simulink model "Main_simulation_davide"  (R2021b)
settings: Solver=FixedStepAuto  StartTime=0.0  StopTime=Time  FixedStep=0.1  RelTol=1e-13  AbsTol=1e-19
values from neighbouring files (symbols this model uses):
  a = 8.6251e06    (= 8625100)    [main_code.m]
  A_BN_0 = eye(3)    [main_code.m]
  A_rw = [1 0 0 1/sqrt(3);         0 1 0 1/sqrt(3) ... (first row only)    [main_code.m]
  A_rw_star = [5/6 -1/6 -1/6;              -1/6  5/6 -1/6 ... (first row only)    [main_code.m]
  acc_m = deg2rad(5)    [main_code.m]
  acc_S = deg2rad(0.25)    [main_code.m]
  c = 2.99792*10^8    (= 299792000)    [main_code.m]
  control = 3    [main_code.m]
  e = 0.1195    [main_code.m]
  G = [gn, gm, gvali, gsvi]    [main_code.m]
  H = [hn, hm, hvali, hsvi]    [main_code.m]
  i = 0.3815    [main_code.m]
  MB = [1; 0.3; 0.3; 0.3]    [main_code.m]
  mr = 1.2*1e-4    (= 0.00012)    [main_code.m]
  mu_P = G * Mt    (= 398527110340000)    [main_code.m]
  omega_0 = [w_0x; w_0y; w_0z]    [main_code.m]
  rho_d_MB = 0.1    [main_code.m]
  rho_d_SP = 0.1    [main_code.m]
  rho_s_MB = 0.5    [main_code.m]
  rho_s_SP = 0.1    [main_code.m]
  sig_b = sig_b^2    [main_code.m]
  sig_n = 0.15*pi/180/3600/sqrt(t_sample)    [main_code.m]
  SP = [3; 0.3; 1; 0.1]    [main_code.m]
  t_sample = 1    [main_code.m]
  theta_0 = 0    [main_code.m]
undefined symbols (not defined in the file or in its folder): theta0
libraries: matrix_library x16, vrlib x10, simulink x3, simulink_extras x1
(part 2 of 4)

== system Main_simulation_davide/Attitude determination/Attitude determination/If Action Subsystem3 ==
  In1 : Inport
  Action Port : ActionPort  ActionPortLabel=if(u1 == u2)
  Out1 : Outport
  wires:
  In1/1 -> Out1/1

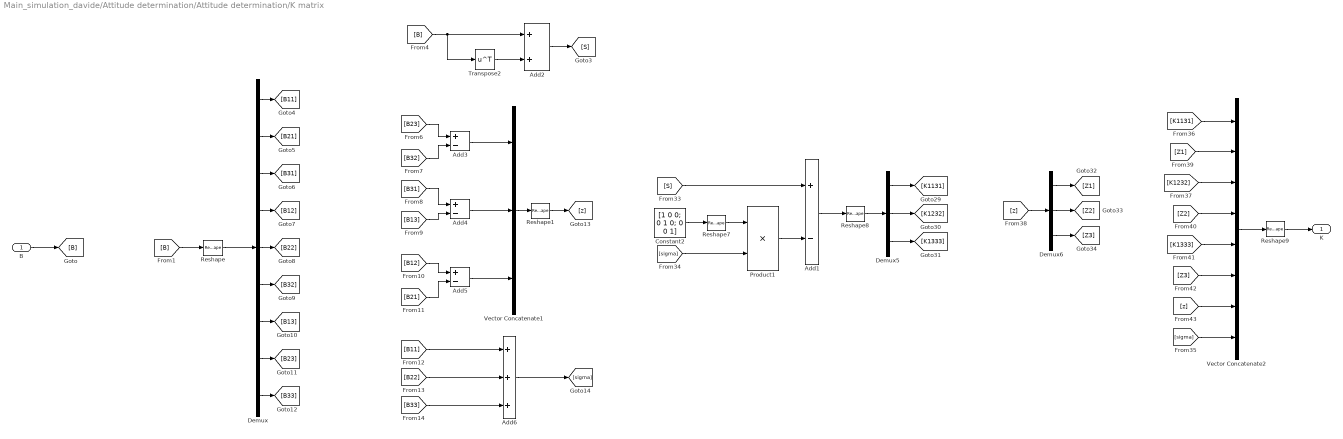
== system Main_simulation_davide/Attitude determination/Attitude determination/K matrix ==
  B : Inport
  Add{1,3..5} (4 alike) : Sum  Inputs=+-
  Add2 : Sum
  Add6 : Sum  Inputs=+++
  Constant2 : Constant  Value=[1 0 0; 0 1 0; 0 0 1]  VectorParams1D=off
  Demux : Demux  Outputs=9
  Demux5 : Demux  Outputs=3
  Demux6 : Demux  Outputs=3
  Product1 : Product
  Reshape : Reshape  OutputDimensionality=Column vector (2-D)
  Reshape1 : Reshape  OutputDimensionality=Column vector (2-D)
  Reshape7 : Reshape  OutputDimensionality=Customize  OutputDimensions=[3,3]
  Reshape8 : Reshape  OutputDimensionality=Column vector (2-D)
  Reshape9 : Reshape  OutputDimensionality=Customize  OutputDimensions=[4,4]
  Transpose2 : Math  Operator=transpose  SaturateOnIntegerOverflow=on
  Vector Concatenate1 : Concatenate  NumInputs=3
  Vector Concatenate2 : Concatenate  NumInputs=8
  K : Outport
  wires:
  Demux/9 -> [B33]
  Demux/3 -> [B31]
  Demux/5 -> [B22]
  Demux/2 -> [B21]
  Demux/8 -> [B23]
  Demux/7 -> [B13]
  Reshape/1 -> Demux/1
  Demux/6 -> [B32]
  Demux/1 -> [B11]
  Demux/4 -> [B12]
  Demux6/3 -> [Z3]
  [B21] -> Add5/2
  [B32] -> Add3/2
  [B33] -> Add6/3
  [B22] -> Add6/2
  [B23] -> Add3/1
  [B12] -> Add5/1
  Add4/1 -> Vector Concatenate1/2
  Transpose2/1 -> Add2/2
  Add5/1 -> Vector Concatenate1/3
  [B31] -> Add4/1
  Vector Concatenate1/1 -> Reshape1/1
  Reshape1/1 -> [z]
  Add6/1 -> [sigma]
  [B13] -> Add4/2
  [B11] -> Add6/1
  Add3/1 -> Vector Concatenate1/1
  [B] -> Transpose2/1, Add2/1
  Demux6/1 -> [Z1]
  Reshape8/1 -> Demux5/1
  Product1/1 -> Add1/2
  [S] -> Add1/1
  Constant2/1 -> Reshape7/1
  [sigma] -> Product1/2
  Add2/1 -> [S]
  Demux6/2 -> [Z2]
  Reshape7/1 -> Product1/1
  Demux5/2 -> [K1232]
  Demux5/3 -> [K1333]
  Demux5/1 -> [K1131]
  Add1/1 -> Reshape8/1
  [z] -> Demux6/1
  Vector Concatenate2/1 -> Reshape9/1
  [K1333] -> Vector Concatenate2/5
  [sigma] -> Vector Concatenate2/8
  [z] -> Vector Concatenate2/7
  [K1131] -> Vector Concatenate2/1
  [K1232] -> Vector Concatenate2/3
  [Z1] -> Vector Concatenate2/2
  [Z3] -> Vector Concatenate2/6
  [Z2] -> Vector Concatenate2/4
  Reshape9/1 -> K/1
  B/1 -> [B]
  [B] -> Reshape/1

== system Main_simulation_davide/Attitude determination/Attitude determination/q to DCM ==
  In1 : Inport
  Add : Sum  Inputs=+-
  Add1 : Sum  Inputs=++-
  Constant : Constant  Value=[1 0 0; 0 1 0; 0 0 1]  VectorParams1D=off
  Demux : Demux
  Gain : Gain  Gain=2
  Gain1 : Gain  Gain=2
  Matrix Multiply : Product  Multiplication=Matrix(*)
  Matrix Multiply2 : Product  Multiplication=Matrix(*)
  Mux : Mux  Inputs=3
  Product : Product
  Product1 : Product
  Reshape : Reshape  OutputDimensionality=Column vector (2-D)
  Reshape1 : Reshape  OutputDimensionality=Customize  OutputDimensions=[3,3]
  Square : Math  Operator=square  SaturateOnIntegerOverflow=on
  Transpose : Math  Operator=transpose  SaturateOnIntegerOverflow=on
  Transpose1 : Math  Operator=transpose  SaturateOnIntegerOverflow=on
  q_cross : Subsystem
  A_BN : Outport
  wires:
  In1/1 -> Demux/1
  Demux/4 -> [q4]
  Demux/1 -> [q1]
  Demux/2 -> [q2]
  Demux/3 -> [q3]
  [q4] -> Square/1
  [q2] -> Mux/2
  [q3] -> Mux/3
  [q1] -> Mux/1
  Mux/1 -> Reshape/1
  Reshape/1 -> [q_vect]
  [q_vect] -> Matrix Multiply/2, Transpose/1
  Transpose/1 -> Matrix Multiply/1
  Matrix Multiply/1 -> Add/2
  Square/1 -> Add/1
  Constant/1 -> Reshape1/1
  Reshape1/1 -> Product1/2
  Product1/1 -> Add1/1
  Matrix Multiply2/1 -> Gain/1
  Gain/1 -> Add1/2
  Transpose1/1 -> Matrix Multiply2/2
  [q_vect] -> Transpose1/1, Matrix Multiply2/1
  Gain1/1 -> Add1/3
  Product/1 -> Gain1/1
  [q4] -> Product/2
  q_cross/1(q_cross) -> Product/1
  Add1/1 -> A_BN/1
  [q_vect] -> q_cross/1(q_vect)
  Add/1 -> Product1/1

== system Main_simulation_davide/Attitude determination/Quaternion error/Q matrix ==
  q_eul : Inport
  Demux : Demux
  Gain{,1..5} (6 alike) : Gain  Gain=-1
  Reshape : Reshape  OutputDimensionality=Customize  OutputDimensions=[4,4]
  Vector Concatenate : Concatenate  NumInputs=16
  Q_eul : Outport
  wires:
  q_eul/1 -> Demux/1
  Demux/1 -> [q1]
  Demux/2 -> [q2]
  Demux/3 -> [q3]
  Demux/4 -> [q4]
  Reshape/1 -> Q_eul/1
  Vector Concatenate/1 -> Reshape/1
  [q4] -> Vector Concatenate/1
  [q3] -> Gain/1
  Gain/1 -> Vector Concatenate/2
  [q2] -> Vector Concatenate/3
  [q1] -> Vector Concatenate/4
  [q3] -> Vector Concatenate/5
  [q4] -> Vector Concatenate/6
  Gain1/1 -> Vector Concatenate/7
  [q1] -> Gain1/1
  [q2] -> Vector Concatenate/8
  [q2] -> Gain2/1
  Gain2/1 -> Vector Concatenate/9
  [q1] -> Vector Concatenate/10
  [q4] -> Vector Concatenate/11
  [q3] -> Vector Concatenate/12
  [q1] -> Gain3/1
  Gain4/1 -> Vector Concatenate/14
  Gain3/1 -> Vector Concatenate/13
  Gain5/1 -> Vector Concatenate/15
  [q2] -> Gain4/1
  [q3] -> Gain5/1
  [q4] -> Vector Concatenate/16

== system Main_simulation_davide/Attitude determination/Sensors/Gyroscopes ==
  note: gyro model: STIM300
  omega : Inport
  Integrator : Integrator
  Mux1 : Mux  Inputs=3
  Mux2 : Mux  Inputs=3
  Reshape : Reshape  OutputDimensionality=Column vector (2-D)
  Reshape1 : Reshape  OutputDimensionality=Column vector (2-D)
  Sum : Sum  Inputs=+++
  "b1 " : RandomNumber  Variance=sig_b  Seed=1  SampleTime=t_sample
  b2 : RandomNumber  Variance=sig_b  Seed=2  SampleTime=t_sample
  b3 : RandomNumber  Variance=sig_b  Seed=3  SampleTime=t_sample
  n1 : RandomNumber  Variance=sig_n  Seed=4  SampleTime=t_sample
  n2 : RandomNumber  Variance=sig_n  Seed=5  SampleTime=t_sample
  n3 : RandomNumber  Variance=sig_n  Seed=6  SampleTime=t_sample
  w_gyro : Outport
  wires:
  Integrator/1 -> Sum/1
  "b1 "/1 -> Mux1/1
  b2/1 -> Mux1/2
  b3/1 -> Mux1/3
  n3/1 -> Mux2/3
  n2/1 -> Mux2/2
  n1/1 -> Mux2/1
  Mux1/1 -> Reshape/1
  Mux2/1 -> Reshape1/1
  omega/1 -> Sum/2
  Reshape/1 -> Integrator/1
  Reshape1/1 -> Sum/3
  Sum/1 -> w_gyro/1

== system Main_simulation_davide/Attitude determination/Sensors/Magnetometer ==
  A_BN : Inport
  b_N : Inport  Port=2
  "Magnetometer " : Subsystem
  b_B computation : Subsystem
  model to reality difference : Subsystem
  b_B : Outport
  wires:
  "Magnetometer "/1(A_BN*_filtered) -> model to reality difference/2(A_BN*), b_B computation/1(A_BN*)
  A_BN/1 -> model to reality difference/1(A_BN), "Magnetometer "/1(A_BN)
  b_N/1 -> b_B computation/2(b_N), model to reality difference/3(b_N)
  b_B computation/1(b_B) -> b_B/1

== system Main_simulation_davide/Attitude determination/Sensors/Sun sensor ==
  note: redwire space, digital sun sensor +/- 64°
  S_N : Inport
  A_BN : Inport  Port=2
  Add : Sum  Inputs=+-
  Add1 : Sum  Inputs=+-
  Constant : Constant  Value=0.25*pi/180
  Constant1 : Constant
  Constant2 : Constant  Value=0.25*pi/180
  Constant3 : Constant  Value=0.25*pi/180
  Discrete Derivative : simulink/Discrete/Discrete Derivative  gainval=1e4  ICPrevScaledInput=0.0  OutMin=[]  OutMax=[]  OutDataType=fixdt(1, 16)  OutScaling=2^-10  DoSatur=off
  Gain : Gain  Gain=-1
  Gain1 : Gain  Gain=-1
  Gain2 : Gain  Gain=-1
  Matrix Multiply : Product  Multiplication=Matrix(*)
  Matrix Multiply1 : Product  Multiplication=Matrix(*)
  Product : Product
  Product1 : Product
  Product2 : Product
  Random Number : RandomNumber  Variance=0.6*pi/180  SampleTime=t_sample
  Random Number1 : RandomNumber  Variance=0.6*pi/180  SampleTime=t_sample
  Random Number2 : RandomNumber  Variance=0.6*pi/180  SampleTime=t_sample
  Reshape : Reshape  OutputDimensionality=Customize  OutputDimensions=[3,3]
  Scope : Scope
  Vector Concatenate : Concatenate  NumInputs=9
  S_B : Outport
  wires:
  S_N/1 -> Matrix Multiply1/2
  Random Number/1 -> Product/2
  Constant/1 -> Product/1
  Matrix Multiply/1 -> Add1/1
  Add1/1 -> Add/1, Discrete Derivative/1, S_B/1
  Constant1/1 -> Vector Concatenate/8, Vector Concatenate/5, Vector Concatenate/1
  Constant2/1 -> Product1/1
  Random Number1/1 -> Product1/2
  Random Number2/1 -> Product2/2
  Constant3/1 -> Product2/1
  Product2/1 -> Vector Concatenate/4, Gain/1
  Gain/1 -> Vector Concatenate/2
  Product1/1 -> Vector Concatenate/3, Gain2/1
  Gain1/1 -> Vector Concatenate/6
  Product/1 -> Gain1/1, Vector Concatenate/9
  Gain2/1 -> Vector Concatenate/7
  Discrete Derivative/1 -> Add1/2
  Reshape/1 -> Matrix Multiply/1
  Vector Concatenate/1 -> Reshape/1
  A_BN/1 -> Matrix Multiply1/1
  Matrix Multiply1/1 -> Add/2, Matrix Multiply/2
  Add/1 -> Scope/1

== system Main_simulation_davide/Control/Slew/Desired attitude ==
  S_N : Inport
  Constant : Constant  Value=0
  Constant1 : Constant
  Constant2 : Constant  Value=0
  Cross Product : matrix_library/Cross Product
      settings: SourceProductBaseCode=SL
  Display : Display
  Display1 : Display
  Dot Product : DotProduct  InputSameDT=on  OutDataTypeStr=Inherit: Inherit via internal rule
  Matrix Multiply : Product  Multiplication=Matrix(*)
  Mux : Mux  Inputs=3
  Reshape : Reshape  OutputDimensionality=Column vector (2-D)
  Reshape1 : Reshape  OutputDimensionality=Customize  OutputDimensions=[3,3]
  Transpose : Math  Operator=transpose  SaturateOnIntegerOverflow=on
  Transpose1 : Math  Operator=transpose  SaturateOnIntegerOverflow=on
  Vector Concatenate : Concatenate  NumInputs=3
  orthonormalization step 1 : Subsystem
  Desired A_BN : Outport
  wires:
  Constant/1 -> Mux/1
  Constant1/1 -> Mux/2
  Constant2/1 -> Mux/3
  Mux/1 -> Reshape/1
  Reshape/1 -> Vector Concatenate/2, Cross Product/2
  S_N/1 -> Dot Product/2, Dot Product/1, Vector Concatenate/1, Cross Product/1
  Vector Concatenate/1 -> Reshape1/1
  Reshape1/1 -> Transpose/1
  Transpose1/1 -> Matrix Multiply/2
  Matrix Multiply/1 -> Display/1
  Dot Product/1 -> Display1/1
  Transpose/1 -> orthonormalization step 1/1(A*(t))
  orthonormalization step 1/1(A_BN*_filtered) -> Transpose1/1, Matrix Multiply/1, Desired A_BN/1
  Cross Product/1 -> Vector Concatenate/3

== system Main_simulation_davide/Control/Slew/Reaction wheel ==
  Mc : Inport
  w : Inport  Port=2
  A : Constant  Value=A_rw
  A_star : Constant  Value=A_rw_star
  Add : Sum  Inputs=--
  Constant : Constant  Value=[0 0 0 0]
  Cross Product : matrix_library/Cross Product
      settings: SourceProductBaseCode=SL
  Cross Product1 : matrix_library/Cross Product
      settings: SourceProductBaseCode=SL
  Gain : Gain  Gain=-1
  Integrator : Integrator  InitialConditionSource=external
  Matrix Multiply{,1..3} (4 alike) : Product  Multiplication=Matrix(*)
  Reshape : Reshape  OutputDimensionality=Column vector (2-D)
  Reshape1 : Reshape  OutputDimensionality=Column vector (2-D)
  Sum : Sum  Inputs=|++
  Mr : Outport
  wires:
  Cross Product1/1 -> Add/2
  [h_r] -> Matrix Multiply3/2
  [A_rw] -> Matrix Multiply3/1
  Matrix Multiply3/1 -> Cross Product1/2
  [omega] -> Cross Product1/1
  Add/1 -> Mr/1
  Matrix Multiply2/1 -> Add/1
  [A_rw] -> Matrix Multiply2/1
  Reshape1/1 -> Sum/2
  Reshape/1 -> Integrator/2
  Constant/1 -> Reshape/1
  Matrix Multiply1/1 -> Matrix Multiply2/2, Integrator/1
  Gain/1 -> Matrix Multiply1/1
  A_star/1 -> Gain/1
  Sum/1 -> Matrix Multiply1/2
  Mc/1 -> Reshape1/1
  Cross Product/1 -> Sum/1
  Matrix Multiply/1 -> Cross Product/2
  w/1 -> Cross Product/1, [omega]
  A/1 -> Matrix Multiply/1, [A_rw]
  Integrator/1 -> Matrix Multiply/2, [h_r]

== system Main_simulation_davide/Control/Target tracking/Reaction wheel ==
  Mc : Inport
  w : Inport  Port=2
  A : Constant  Value=A_rw
  A_star : Constant  Value=A_rw_star
  Add : Sum  Inputs=--
  Constant : Constant  Value=[0 0 0 0]
  Cross Product : matrix_library/Cross Product
      settings: SourceProductBaseCode=SL
  Cross Product1 : matrix_library/Cross Product
      settings: SourceProductBaseCode=SL
  Gain : Gain  Gain=-1
  Integrator : Integrator  InitialConditionSource=external
  Matrix Multiply{,1..3} (4 alike) : Product  Multiplication=Matrix(*)
  Reshape : Reshape  OutputDimensionality=Column vector (2-D)
  Reshape1 : Reshape  OutputDimensionality=Column vector (2-D)
  Sum : Sum  Inputs=|++
  Mr : Outport
  wires:
  Cross Product1/1 -> Add/2
  [h_r] -> Matrix Multiply3/2
  [A_rw] -> Matrix Multiply3/1
  Matrix Multiply3/1 -> Cross Product1/2
  [omega] -> Cross Product1/1
  Add/1 -> Mr/1
  Matrix Multiply2/1 -> Add/1
  [A_rw] -> Matrix Multiply2/1
  Reshape1/1 -> Sum/2
  Reshape/1 -> Integrator/2
  Constant/1 -> Reshape/1
  Matrix Multiply1/1 -> Matrix Multiply2/2, Integrator/1
  Gain/1 -> Matrix Multiply1/1
  A_star/1 -> Gain/1
  Sum/1 -> Matrix Multiply1/2
  Mc/1 -> Reshape1/1
  Cross Product/1 -> Sum/1
  Matrix Multiply/1 -> Cross Product/2
  w/1 -> Cross Product/1, [omega]
  A/1 -> Matrix Multiply/1, [A_rw]
  Integrator/1 -> Matrix Multiply/2, [h_r]

== system Main_simulation_davide/Enviroment/Magnetic field/b_B ==
  A_BN : Inport
  R : Inport  Port=2
  r_LVLH : Inport  Port=3
  Clock : Clock
  Constant3 : Constant  Value=G
  Constant4 : Constant  Value=H
  MATLAB Function : MATLAB Function  TreatAsAtomicUnit=on
  MatrixMultiply : Product  Multiplication=Matrix(*)
  Reshape1 : Reshape  OutputDimensionality=Column vector (2-D)
  b_B : Outport
  b_N : Outport  Port=2
  wires:
  MatrixMultiply/1 -> b_B/1
  A_BN/1 -> [A_BN]
  [A_BN] -> MatrixMultiply/1
  r_LVLH/1 -> MATLAB Function/1(r_LVLH)
  R/1 -> MATLAB Function/2(r)
  Clock/1 -> MATLAB Function/3(t)
  MATLAB Function/1(b_N) -> Reshape1/1
  Constant3/1 -> MATLAB Function/4(G)
  Constant4/1 -> MATLAB Function/5(H)
  Reshape1/1 -> b_N/1, MatrixMultiply/2

== system Main_simulation_davide/Enviroment/Magnetic field/parasitic torque ==
  Constant : Constant  Value=0.01
  Constant1 : Constant  Value=0.05
  Constant2 : Constant  Value=0.01
  Mux : Mux  Inputs=3
  Reshape : Reshape  OutputDimensionality=Column vector (2-D)
  m_par : Outport
  wires:
  Constant/1 -> Mux/1
  Constant1/1 -> Mux/2
  Constant2/1 -> Mux/3
  Mux/1 -> Reshape/1
  Reshape/1 -> m_par/1

== system Main_simulation_davide/Enviroment/Solar radiation/Areas ==
  MB : Inport
  Demux : Demux
  Mux : Mux  Inputs=3
  Product1 : Product
  Product2 : Product
  Product4 : Product
  Terminator : Terminator
  A_vect : Outport
  wires:
  Product2/1 -> Mux/2  "a*h"
  Product4/1 -> Mux/1  "b*h"
  MB/1 -> Demux/1
  Product1/1 -> Mux/3  "a*b"
  Demux/1 -> Terminator/1
  Demux/2 -> [a]
  Demux/3 -> [b]
  Demux/4 -> [h]
  [b] -> Product4/1
  [h] -> Product4/2
  [h] -> Product2/2
  [b] -> Product1/2
  [a] -> Product2/1
  [a] -> Product1/1
  Mux/1 -> A_vect/1

== system Main_simulation_davide/Enviroment/Solar radiation/Areas_SP ==
  SP : Inport
  Demux : Demux
  Product1 : Product
  Terminator : Terminator
  Terminator1 : Terminator
  A_vect : Outport
  wires:
  [a] -> Product1/1
  [b] -> Product1/2
  Demux/4 -> Terminator1/1
  Demux/3 -> [b]
  Demux/2 -> [a]
  Demux/1 -> Terminator/1
  Product1/1 -> A_vect/1  "a*b"
  SP/1 -> Demux/1

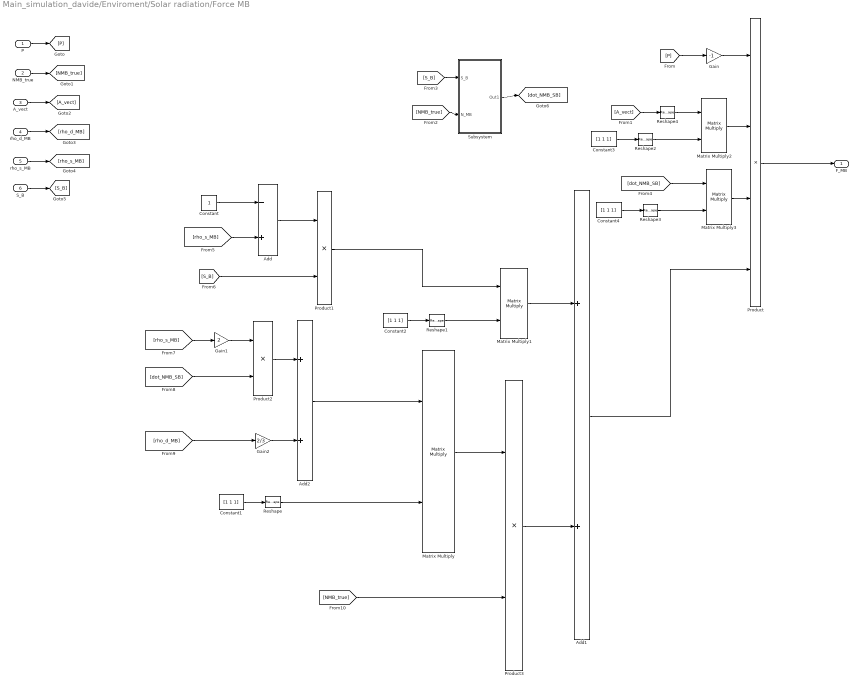
== system Main_simulation_davide/Enviroment/Solar radiation/Force MB ==
  P : Inport
  NMB_true : Inport  Port=2
  A_vect : Inport  Port=3
  rho_d_MB : Inport  Port=4
  rho_s_MB : Inport  Port=5
  S_B : Inport  Port=6
  Add : Sum  Inputs=-+
  Add1 : Sum
  Add2 : Sum
  Constant : Constant
  Constant{1..4} (4 alike) : Constant  Value=[1 1 1]
  Gain : Gain  Gain=-1
  Gain1 : Gain  Gain=2
  Gain2 : Gain  Gain=2/3
  Matrix Multiply{,1..3} (4 alike) : Product  Multiplication=Matrix(*)
  Product : Product  Inputs=4
  Product1 : Product
  Product2 : Product
  Product3 : Product
  Reshape{,1..3} (4 alike) : Reshape  OutputDimensionality=Row vector (2-D)
  Reshape4 : Reshape  OutputDimensionality=Column vector (2-D)
  Subsystem : Subsystem
  F_MB : Outport
  wires:
  Product/1 -> F_MB/1
  P/1 -> [P]
  NMB_true/1 -> [NMB_true]
  A_vect/1 -> [A_vect]
  rho_d_MB/1 -> [rho_d_MB]
  rho_s_MB/1 -> [rho_s_MB]
  S_B/1 -> [S_B]
  [P] -> Gain/1
  Gain/1 -> Product/1
  [NMB_true] -> Subsystem/2(N_MB)
  [S_B] -> Subsystem/1(S_B)
  Subsystem/1(Out1) -> [dot_NMB_SB]
  [rho_s_MB] -> Add/2
  Constant/1 -> Add/1
  Add/1 -> Product1/1
  [S_B] -> Product1/2
  [rho_s_MB] -> Gain1/1
  [dot_NMB_SB] -> Product2/2
  Gain1/1 -> Product2/1
  Product2/1 -> Add2/1
  Gain2/1 -> Add2/2
  [rho_d_MB] -> Gain2/1
  [NMB_true] -> Product3/2
  Product3/1 -> Add1/2
  Add1/1 -> Product/4
  Constant1/1 -> Reshape/1
  Matrix Multiply/1 -> Product3/1
  Add2/1 -> Matrix Multiply/1
  Reshape/1 -> Matrix Multiply/2
  Matrix Multiply1/1 -> Add1/1
  Product1/1 -> Matrix Multiply1/1
  Constant2/1 -> Reshape1/1
  Reshape1/1 -> Matrix Multiply1/2
  Reshape2/1 -> Matrix Multiply2/2
  Constant3/1 -> Reshape2/1
  Reshape3/1 -> Matrix Multiply3/2
  Constant4/1 -> Reshape3/1
  [A_vect] -> Reshape4/1
  Reshape4/1 -> Matrix Multiply2/1
  [dot_NMB_SB] -> Matrix Multiply3/1
  Matrix Multiply3/1 -> Product/3
  Matrix Multiply2/1 -> Product/2

== system Main_simulation_davide/Enviroment/Solar radiation/Force SP ==
  P : Inport
  NSP_true : Inport  Port=2
  A_vect_SP : Inport  Port=3
  rho_d_SP : Inport  Port=4
  rho_s_SP : Inport  Port=5
  S_B : Inport  Port=6
  Add : Sum  Inputs=+-
  Add1 : Sum
  Add2 : Sum
  Constant : Constant
  Dot Product : DotProduct  InputSameDT=on  OutDataTypeStr=Inherit: Inherit via internal rule
  Dot Product1 : DotProduct  InputSameDT=on  OutDataTypeStr=Inherit: Inherit via internal rule
  Gain : Gain  Gain=-1
  Gain1 : Gain  Gain=2
  Gain2 : Gain  Gain=2/3
  Product : Product  Inputs=4
  Product1 : Product
  Product2 : Product
  Product3 : Product
  Reshape : Reshape  OutputDimensionality=Row vector (2-D)
  Transpose : Math  Operator=transpose  SaturateOnIntegerOverflow=on
  F_SP : Outport
  wires:
  P/1 -> [P]
  NSP_true/1 -> [NSP_true]
  A_vect_SP/1 -> [A_vect_SP]
  rho_d_SP/1 -> [rho_d_SP]
  rho_s_SP/1 -> [rho_s_SP]
  S_B/1 -> [S_B]
  Product/1 -> Reshape/1
  [P] -> Gain/1
  Gain/1 -> Product/1
  [A_vect_SP] -> Product/2
  Dot Product/1 -> Product/3
  [S_B] -> Dot Product/2
  [NSP_true] -> Dot Product/1
  Constant/1 -> Add/1
  [rho_s_SP] -> Add/2
  Add/1 -> Product1/1
  [S_B] -> Product1/2
  [rho_s_SP] -> Gain1/1
  [NSP_true] -> Dot Product1/1
  [S_B] -> Dot Product1/2
  Dot Product1/1 -> Product2/2
  Gain1/1 -> Product2/1
  Product2/1 -> Add1/1
  [rho_d_SP] -> Gain2/1
  Gain2/1 -> Add1/2
  [NSP_true] -> Transpose/1
  Add1/1 -> Product3/1
  Product1/1 -> Add2/1
  Product3/1 -> Add2/2
  Transpose/1 -> Product3/2
  Add2/1 -> Product/4
  Reshape/1 -> F_SP/1

== system Main_simulation_davide/Enviroment/Solar radiation/Pressure ==
  Constant6 : Constant  Value=1358
  Constant7 : Constant  Value=c
  Product8 : Product
  Reciprocal : Product  Inputs=/
  P : Outport
  wires:
  Constant6/1 -> Product8/1
  Reciprocal/1 -> Product8/2
  Product8/1 -> P/1
  Constant7/1 -> Reciprocal/1

== system Main_simulation_davide/Enviroment/Solar radiation/S_B dot N_MB ==
  N_MB : Inport
  S_B : Inport  Port=2
  Constant3 : Constant  Value=[1, 1, 1, 1, 1, 1]  VectorParams1D=off
  Demux : Demux  Outputs=6
  If : If
  If Action Subsystem : Subsystem  TreatAsAtomicUnit=on
  If Action Subsystem1 : Subsystem  TreatAsAtomicUnit=on
  If Action Subsystem2 : Subsystem  TreatAsAtomicUnit=on
  If Action Subsystem3 : Subsystem  TreatAsAtomicUnit=on
  If Action Subsystem4 : Subsystem  TreatAsAtomicUnit=on
  If Action Subsystem5 : Subsystem  TreatAsAtomicUnit=on
  If1 : If
  If2 : If
  Matrix Multiply5 : Product  Multiplication=Matrix(*)
  Merge{,1..5} (6 alike) : Merge
  Mux : Mux  Inputs=3
  Product10 : Product
  Reshape{,1..4,12} (6 alike) : Reshape  OutputDimensionality=Column vector (2-D)
  Reshape11 : Reshape  OutputDimensionality=Row vector (2-D)
  Reshape5 : Reshape  OutputDimensionality=Customize  OutputDimensions=[3,3]
  Sum of Elements : Sum  Inputs=+  CollapseMode=Specified dimension  CollapseDim=2
  Terminator1 : Terminator
  Terminator2 : Terminator
  Terminator3 : Terminator
  Transpose : Math  Operator=transpose  SaturateOnIntegerOverflow=on
  Vector Concatenate : Concatenate  NumInputs=3
  MB_illuminated : Outport
  pointer : Outport  Port=2
  wires:
  Reshape12/1 -> Matrix Multiply5/1
  Matrix Multiply5/1 -> Transpose/1
  Product10/1 -> Sum of Elements/1
  Reshape11/1 -> Matrix Multiply5/2
  Constant3/1 -> Reshape11/1
  S_B/1 -> Reshape12/1
  Sum of Elements/1 -> Reshape/1
  Reshape/1 -> Demux/1
  Demux/1 -> If/1
  If/1 -> If Action Subsystem/Action
  If/2 -> If Action Subsystem3/Action
  N_MB/1 -> [N_MB]
  [N_MB] -> Product10/2
  [N_MB] -> If Action Subsystem/1(NMB)
  Demux/4 -> Terminator1/1
  Demux/5 -> Terminator2/1
  Demux/6 -> Terminator3/1
  Demux/2 -> If1/1
  If1/1 -> If Action Subsystem1/Action
  [N_MB] -> If Action Subsystem3/1(NMB)
  [N_MB] -> If Action Subsystem1/1(NMB)
  If1/2 -> If Action Subsystem4/Action
  [N_MB] -> If Action Subsystem4/1(NMB)
  If Action Subsystem3/1(-x) -> Merge/2
  If Action Subsystem/1(x) -> Merge/1
  If Action Subsystem1/1(y) -> Merge1/1
  If Action Subsystem2/1(z) -> Merge2/1
  If Action Subsystem5/1(-z) -> Merge2/2
  Demux/3 -> If2/1
  If2/1 -> If Action Subsystem2/Action
  If2/2 -> If Action Subsystem5/Action
  [N_MB] -> If Action Subsystem2/1(NMB)
  [N_MB] -> If Action Subsystem5/1(NMB)
  Merge/1 -> Reshape1/1
  Merge1/1 -> Reshape2/1
  Merge2/1 -> Reshape3/1
  Reshape1/1 -> Vector Concatenate/1
  Reshape2/1 -> Vector Concatenate/2
  Reshape3/1 -> Vector Concatenate/3
  Vector Concatenate/1 -> Reshape5/1
  If Action Subsystem4/1(-y) -> Merge1/2
  If Action Subsystem/2(pointer) -> Merge4/1
  If Action Subsystem3/2(pointer) -> Merge4/2
  If Action Subsystem1/2(pointer) -> Merge5/1
  If Action Subsystem4/2(pointer) -> Merge5/2
  If Action Subsystem2/2(pointer) -> Merge3/1
  If Action Subsystem5/2(pointer) -> Merge3/2
  Merge4/1 -> Mux/1
  Merge5/1 -> Mux/2
  Merge3/1 -> Mux/3
  Mux/1 -> Reshape4/1
  Reshape4/1 -> pointer/1
  Reshape5/1 -> MB_illuminated/1
  Transpose/1 -> Product10/1

== system Main_simulation_davide/Enviroment/Solar radiation/S_B dot N_SP ==
  N_SP : Inport
  S_B : Inport  Port=2
  Constant3 : Constant  Value=[1, 1]
  Demux : Demux  Outputs=2
  If : If
  If Action Subsystem : Subsystem  TreatAsAtomicUnit=on
  If Action Subsystem1 : Subsystem  TreatAsAtomicUnit=on
  If1 : If
  Matrix Multiply5 : Product  Multiplication=Matrix(*)
  Merge : Merge
  Merge1 : Merge
  Product10 : Product
  Reshape11 : Reshape  OutputDimensionality=Row vector (2-D)
  Reshape12 : Reshape  OutputDimensionality=Column vector (2-D)
  Sum of Elements : Sum  Inputs=+  CollapseMode=Specified dimension  CollapseDim=2
  Terminator : Terminator
  Terminator1 : Terminator
  Transpose : Math  Operator=transpose  SaturateOnIntegerOverflow=on
  SP_illuminated : Outport
  pointer : Outport  Port=2
  wires:
  [N_SP] -> Product10/2
  N_SP/1 -> [N_SP]
  Sum of Elements/1 -> Demux/1
  S_B/1 -> Reshape12/1
  Constant3/1 -> Reshape11/1
  Reshape11/1 -> Matrix Multiply5/2
  Product10/1 -> Sum of Elements/1
  Matrix Multiply5/1 -> Transpose/1
  Reshape12/1 -> Matrix Multiply5/1
  Transpose/1 -> Product10/1
  Demux/1 -> If/1
  If/1 -> If Action Subsystem/Action
  Demux/2 -> If1/1
  [N_SP] -> If Action Subsystem/1(N_SP)
  [N_SP] -> If Action Subsystem1/1(N_SP)
  If1/1 -> If Action Subsystem1/Action
  If1/2 -> Terminator/1
  If/2 -> Terminator1/1
  If Action Subsystem/1(true_NSP) -> Merge/1
  If Action Subsystem1/1(true_NSP) -> Merge/2
  If Action Subsystem/2(pointer) -> Merge1/1
  If Action Subsystem1/2(pointer) -> Merge1/2
  Merge/1 -> SP_illuminated/1
  Merge1/1 -> pointer/1

== system Main_simulation_davide/Enviroment/Solar radiation/Sun position ==
  A_B_N : Inport
  Clock : Clock
  Constant : Constant  Value=2*pi
  Constant1 : Constant  Value=365*24*60*60
  Constant2 : Constant  Value=23.45
  Degrees to Radians : simulink_extras/Transformations/Degrees to Radians
  MatrixMultiply : Product  Multiplication=Matrix(*)
  Mux : Mux  Inputs=3
  Product{,1..3} (4 alike) : Product
  Reciprocal : Product  Inputs=1
  Reshape : Reshape  OutputDimensionality=Column vector (2-D)
  Sin : Trigonometry  Operator=cos
  Sin1 : Trigonometry
  Sin2 : Trigonometry  Operator=cos
  Sin3 : Trigonometry
  S_B : Outport
  S_N : Outport  Port=2
  wires:
  Product3/1 -> Mux/3
  Degrees to Radians/1 -> Sin3/1, Sin2/1
  Constant1/1 -> Reciprocal/1
  Sin2/1 -> Product2/2
  Product/1 -> Product1/1  "n"
  Constant2/1 -> Degrees to Radians/1
  Product1/1 -> Sin/1, Sin1/1  "n*t"
  Product2/1 -> Mux/2
  Sin3/1 -> Product3/2
  Clock/1 -> Product1/2
  Sin1/1 -> Product3/1, Product2/1
  Constant/1 -> Product/1
  Sin/1 -> Mux/1
  Reciprocal/1 -> Product/2
  Mux/1 -> Reshape/1
  A_B_N/1 -> MatrixMultiply/1
  MatrixMultiply/1 -> S_B/1
  Reshape/1 -> S_N/1, MatrixMultiply/2

== system Main_simulation_davide/Enviroment/Solar radiation/Torque arm MB ==
  note: creo il vettore somma che ha per colonna i raggi vettori che collegano il CM del MB con i centri illuminati delle facce nel caso che il sole sia nelle 4 posizioni.
  MB : Inport
  A_vect : Inport  Port=2
  S_B : Inport  Port=3
  pointer : Inport  Port=4
  Demux : Demux  Outputs=3
  Reshape : Reshape  OutputDimensionality=Customize  OutputDimensions=[3,3]
  Transpose : Math  Operator=transpose  SaturateOnIntegerOverflow=on
  Vector Concatenate : Concatenate  NumInputs=3
  creazione raggi vettore tra CM MB e centro facce illuminate della faccia che ha come normale l'asse i : Subsystem
  creazione raggi vettore tra CM MB e centro facce illuminate della faccia che ha come normale l'asse j : Subsystem
  creazione raggi vettore tra CM MB e centro facce illuminate della faccia che ha come normale l'asse k : Subsystem
  dist : Outport
  wires:
  pointer/1 -> Demux/1
  [x] -> creazione raggi vettore tra CM MB e centro facce illuminate della faccia che ha come normale l'asse i/4(pointer)
  [A_vect] -> creazione raggi vettore tra CM MB e centro facce illuminate della faccia che ha come normale l'asse i/3(A_vect)
  [MB] -> creazione raggi vettore tra CM MB e centro facce illuminate della faccia che ha come normale l'asse k/2(MB)
  [y] -> creazione raggi vettore tra CM MB e centro facce illuminate della faccia che ha come normale l'asse j/4(pointer)
  S_B/1 -> [S_B]
  [A_vect] -> creazione raggi vettore tra CM MB e centro facce illuminate della faccia che ha come normale l'asse k/3(A_vect)
  [MB] -> creazione raggi vettore tra CM MB e centro facce illuminate della faccia che ha come normale l'asse j/2(MB)
  A_vect/1 -> [A_vect]
  MB/1 -> [MB]
  [MB] -> creazione raggi vettore tra CM MB e centro facce illuminate della faccia che ha come normale l'asse i/2(MB)
  Reshape/1 -> Transpose/1
  Transpose/1 -> dist/1
  [S_B] -> creazione raggi vettore tra CM MB e centro facce illuminate della faccia che ha come normale l'asse k/1(S_B)
  Demux/1 -> [x]
  Demux/3 -> [z]
  [S_B] -> creazione raggi vettore tra CM MB e centro facce illuminate della faccia che ha come normale l'asse j/1(S_B)
  [z] -> creazione raggi vettore tra CM MB e centro facce illuminate della faccia che ha come normale l'asse k/4(pointer)
  Vector Concatenate/1 -> Reshape/1  "vectors x, y, z"
  [A_vect] -> creazione raggi vettore tra CM MB e centro facce illuminate della faccia che ha come normale l'asse j/3(A_vect)
  [S_B] -> creazione raggi vettore tra CM MB e centro facce illuminate della faccia che ha come normale l'asse i/1(S_B)
  Demux/2 -> [y]
  creazione raggi vettore tra CM MB e centro facce illuminate della faccia che ha come normale l'asse k/1(Out1) -> Vector Concatenate/3
  creazione raggi vettore tra CM MB e centro facce illuminate della faccia che ha come normale l'asse j/1(Out1) -> Vector Concatenate/2
  creazione raggi vettore tra CM MB e centro facce illuminate della faccia che ha come normale l'asse i/1(Out1) -> Vector Concatenate/1

== system Main_simulation_davide/Enviroment/Solar radiation/Torque arm SP ==
  SP : Inport
  A_vect_SP : Inport  Port=2
  S_B : Inport  Port=3
  pointer_SP : Inport  Port=4
  r_SP1 : Inport  Port=5
  r_SP2 : Inport  Port=6
  Add : Sum
  Add1 : Sum
  Reshape : Reshape  OutputDimensionality=Customize  OutputDimensions=[2,3]
  Vector Concatenate : Concatenate
  creazione raggi vettore tra CM SP e centro facce illuminate della faccia che ha come normale l'asse j : Subsystem
  distance : Outport
  wires:
  Reshape/1 -> distance/1
  SP/1 -> [SP]
  A_vect_SP/1 -> [A_vect_SP]
  S_B/1 -> [S_B]
  pointer_SP/1 -> [pointer_SP]
  r_SP1/1 -> [r_SP1]
  r_SP2/1 -> [r_SP2]
  [S_B] -> creazione raggi vettore tra CM SP e centro facce illuminate della faccia che ha come normale l'asse j/1(S_B)
  [SP] -> creazione raggi vettore tra CM SP e centro facce illuminate della faccia che ha come normale l'asse j/2(SP)
  [A_vect_SP] -> creazione raggi vettore tra CM SP e centro facce illuminate della faccia che ha come normale l'asse j/3(A_vect)
  [pointer_SP] -> creazione raggi vettore tra CM SP e centro facce illuminate della faccia che ha come normale l'asse j/4(pointer)
  creazione raggi vettore tra CM SP e centro facce illuminate della faccia che ha come normale l'asse j/1(distance) -> [distance]
  Vector Concatenate/1 -> Reshape/1
  Add/1 -> Vector Concatenate/1
  [distance] -> Add/1
  [r_SP1] -> Add/2
  [r_SP2] -> Add1/2
  [distance] -> Add1/1
  Add1/1 -> Vector Concatenate/2

== system Main_simulation_davide/Kinematics/DCM to quaternion/Case 1 ==
  A11 : Inport
  A22 : Inport  Port=2
  A33 : Inport  Port=3
  Add : Sum  Inputs=++--
  Constant : Constant
  Gain : Gain  Gain=1/2
  Sqrt : Sqrt  SaturateOnIntegerOverflow=on
  q1 : Outport
  wires:
  A22/1 -> Add/3
  A11/1 -> Add/2
  A33/1 -> Add/4
  Constant/1 -> Add/1
  Add/1 -> Sqrt/1
  Sqrt/1 -> Gain/1
  Gain/1 -> q1/1

== system Main_simulation_davide/Kinematics/DCM to quaternion/Case 2 ==
  A11 : Inport
  A22 : Inport  Port=2
  A33 : Inport  Port=3
  Add : Sum  Inputs=+-+-
  Constant : Constant
  Gain : Gain  Gain=1/2
  Sqrt : Sqrt  SaturateOnIntegerOverflow=on
  q2 : Outport
  wires:
  Gain/1 -> q2/1
  Sqrt/1 -> Gain/1
  Add/1 -> Sqrt/1
  Constant/1 -> Add/1
  A33/1 -> Add/4
  A11/1 -> Add/2
  A22/1 -> Add/3

== system Main_simulation_davide/Kinematics/DCM to quaternion/Case 3 ==
  A11 : Inport
  A22 : Inport  Port=2
  A33 : Inport  Port=3
  Add : Sum  Inputs=+--+
  Constant : Constant
  Gain : Gain  Gain=1/2
  Sqrt : Sqrt  SaturateOnIntegerOverflow=on
  q3 : Outport
  wires:
  A22/1 -> Add/3
  A11/1 -> Add/2
  A33/1 -> Add/4
  Constant/1 -> Add/1
  Add/1 -> Sqrt/1
  Sqrt/1 -> Gain/1
  Gain/1 -> q3/1

== system Main_simulation_davide/Kinematics/DCM to quaternion/Case 4 ==
  A11 : Inport
  A22 : Inport  Port=2
  A33 : Inport  Port=3
  Add : Sum  Inputs=++++
  Constant : Constant
  Gain : Gain  Gain=1/2
  Sqrt : Sqrt  SaturateOnIntegerOverflow=on
  q4 : Outport
  wires:
  Gain/1 -> q4/1
  Sqrt/1 -> Gain/1
  Add/1 -> Sqrt/1
  Constant/1 -> Add/1
  A33/1 -> Add/4
  A11/1 -> Add/2
  A22/1 -> Add/3

== system Main_simulation_davide/Kinematics/DCM to quaternion/If Action Subsystem ==
  In2 : Inport
  In1 : Inport  Port=2
  Action Port : ActionPort  ActionPortLabel=if(u1 == u2)
  Add : Sum
  Add1 : Sum
  Add2 : Sum  Inputs=+-
  Demux : Demux  Outputs=6
  Gain : Gain  Gain=4
  Mux : Mux
  Product : Product
  Product1 : Product
  Product2 : Product
  Reciprocal : Product  Inputs=/
  Reshape : Reshape  OutputDimensionality=Column vector (2-D)
  q_vect1 : Outport
  wires:
  In1/1 -> Demux/1
  In2/1 -> [q1]
  Mux/1 -> Reshape/1
  Reshape/1 -> q_vect1/1
  [q1] -> Mux/1
  Demux/3 -> [A12]
  Demux/2 -> [A31]
  Demux/1 -> [A21]
  Demux/6 -> [A23]
  Demux/5 -> [A13]
  Demux/4 -> [A32]
  [q1] -> Gain/1
  Gain/1 -> Reciprocal/1
  Reciprocal/1 -> [q1_div]
  Add/1 -> Product/1
  [A21] -> Add/2
  [A12] -> Add/1
  [q1_div] -> Product/2
  Product/1 -> [q2]
  Product1/1 -> [q3]
  [q1_div] -> Product1/2
  [A13] -> Add1/1
  [A31] -> Add1/2
  Add1/1 -> Product1/1
  Add2/1 -> Product2/1
  [A32] -> Add2/2
  [A23] -> Add2/1
  [q1_div] -> Product2/2
  Product2/1 -> [q4]
  [q2] -> Mux/2
  [q3] -> Mux/3
  [q4] -> Mux/4

== system Main_simulation_davide/Kinematics/DCM to quaternion/If Action Subsystem1 ==
  In2 : Inport
  In1 : Inport  Port=2
  Action Port : ActionPort  ActionPortLabel=elseif(u1 == u3)
  Add : Sum
  Add1 : Sum  Inputs=-+
  Add2 : Sum
  Demux : Demux  Outputs=6
  Gain : Gain  Gain=4
  Mux : Mux
  Product : Product
  Product1 : Product
  Product2 : Product
  Reciprocal : Product  Inputs=/
  Reshape : Reshape  OutputDimensionality=Column vector (2-D)
  q_vect2 : Outport
  wires:
  [q4] -> Mux/4
  [q3] -> Mux/3
  [q2] -> Mux/2
  Product2/1 -> [q3]
  [q2_div] -> Product2/2
  [A23] -> Add2/1
  [A32] -> Add2/2
  Add2/1 -> Product2/1
  Add1/1 -> Product1/1
  [A31] -> Add1/2
  [A13] -> Add1/1
  [q2_div] -> Product1/2
  Product1/1 -> [q4]
  Product/1 -> [q1]
  [q2_div] -> Product/2
  [A12] -> Add/1
  [A21] -> Add/2
  Add/1 -> Product/1
  Reciprocal/1 -> [q2_div]
  Gain/1 -> Reciprocal/1
  [q2] -> Gain/1
  Demux/4 -> [A32]
  Demux/5 -> [A13]
  Demux/6 -> [A23]
  Demux/1 -> [A21]
  Demux/2 -> [A31]
  Demux/3 -> [A12]
  [q1] -> Mux/1
  Reshape/1 -> q_vect2/1
  Mux/1 -> Reshape/1
  In2/1 -> [q2]
  In1/1 -> Demux/1

== system Main_simulation_davide/Kinematics/DCM to quaternion/If Action Subsystem2 ==
  In2 : Inport
  In1 : Inport  Port=2
  Action Port : ActionPort  ActionPortLabel=elseif( u1 == u4)
  Add : Sum  Inputs=+-
  Add1 : Sum
  Add2 : Sum  Inputs=+-
  Demux : Demux  Outputs=6
  Gain : Gain  Gain=4
  Mux : Mux
  Product : Product
  Product1 : Product
  Product2 : Product
  Reciprocal : Product  Inputs=/
  Reshape : Reshape  OutputDimensionality=Column vector (2-D)
  q_vect3 : Outport
  wires:
  In1/1 -> Demux/1
  In2/1 -> [q3]
  Mux/1 -> Reshape/1
  Reshape/1 -> q_vect3/1
  [q1] -> Mux/1
  Demux/3 -> [A12]
  Demux/2 -> [A31]
  Demux/1 -> [A21]
  Demux/6 -> [A23]
  Demux/5 -> [A13]
  Demux/4 -> [A32]
  [q3] -> Gain/1
  Gain/1 -> Reciprocal/1
  Reciprocal/1 -> [q3_div]
  Add/1 -> Product/1
  [A21] -> Add/2
  [A12] -> Add/1
  [q3_div] -> Product/2
  Product/1 -> [q4]
  Product1/1 -> [q1]
  [q3_div] -> Product1/2
  [A13] -> Add1/1
  [A31] -> Add1/2
  Add1/1 -> Product1/1
  Add2/1 -> Product2/1
  [A32] -> Add2/2
  [A23] -> Add2/1
  [q3_div] -> Product2/2
  Product2/1 -> [q2]
  [q2] -> Mux/2
  [q3] -> Mux/3
  [q4] -> Mux/4

== system Main_simulation_davide/Kinematics/DCM to quaternion/If Action Subsystem3 ==
  In2 : Inport
  In1 : Inport  Port=2
  Action Port : ActionPort  ActionPortLabel=elseif( u1 == u5)
  Add : Sum  Inputs=+-
  Add1 : Sum  Inputs=-+
  Add2 : Sum  Inputs=+-
  Demux : Demux  Outputs=6
  Gain : Gain  Gain=4
  Mux : Mux
  Product : Product
  Product1 : Product
  Product2 : Product
  Reciprocal : Product  Inputs=/
  Reshape : Reshape  OutputDimensionality=Column vector (2-D)
  q_vect4 : Outport
  wires:
  [q4] -> Mux/4
  [q3] -> Mux/3
  [q2] -> Mux/2
  Product2/1 -> [q1]
  [q4_div] -> Product2/2
  [A23] -> Add2/1
  [A32] -> Add2/2
  Add2/1 -> Product2/1
  Add1/1 -> Product1/1
  [A31] -> Add1/2
  [A13] -> Add1/1
  [q4_div] -> Product1/2
  Product1/1 -> [q2]
  Product/1 -> [q3]
  [q4_div] -> Product/2
  [A12] -> Add/1
  [A21] -> Add/2
  Add/1 -> Product/1
  Reciprocal/1 -> [q4_div]
  Gain/1 -> Reciprocal/1
  [q4] -> Gain/1
  Demux/4 -> [A32]
  Demux/5 -> [A13]
  Demux/6 -> [A23]
  Demux/1 -> [A21]
  Demux/2 -> [A31]
  Demux/3 -> [A12]
  [q1] -> Mux/1
  Reshape/1 -> q_vect4/1
  Mux/1 -> Reshape/1
  In2/1 -> [q4]
  In1/1 -> Demux/1

== system Main_simulation_davide/Kinematics/q to DCM/q cross ==
  q_vec : Inport
  Demux : Demux  Outputs=3
  Gain : Gain  Gain=-1
  Gain1 : Gain  Gain=-1
  Gain2 : Gain  Gain=-1
  Ground : Ground
  Reshape : Reshape  OutputDimensionality=Customize  OutputDimensions=[3,3]
  Vector Concatenate : Concatenate  NumInputs=9
  q cross : Outport
  wires:
  Reshape/1 -> q cross/1
  Vector Concatenate/1 -> Reshape/1
  Ground/1 -> Vector Concatenate/9, Vector Concatenate/5, Vector Concatenate/1
  q_vec/1 -> Demux/1
  Demux/1 -> [q1]
  Demux/2 -> [q2]
  Demux/3 -> [q3]
  [q3] -> Vector Concatenate/2
  Gain/1 -> Vector Concatenate/3
  [q2] -> Gain/1
  Gain1/1 -> Vector Concatenate/4
  [q3] -> Gain1/1
  [q1] -> Vector Concatenate/6
  [q2] -> Vector Concatenate/7
  [q1] -> Gain2/1
  Gain2/1 -> Vector Concatenate/8

== system Main_simulation_davide/Relative attitude/A_LN/inclination matrix ==
  i : Inport
  Constant{1..4} (4 alike) : Constant  Value=0
  Constant5 : Constant
  Cos : Trigonometry  Operator=cos
  Cos1 : Trigonometry
  Cos2 : Trigonometry  Operator=cos
  Cos3 : Trigonometry
  Multiply : Gain  Gain=-1
  Mux : Mux  Inputs=3
  Mux1 : Mux  Inputs=3
  Mux2 : Mux  Inputs=3
  Reshape : Reshape  OutputDimensionality=Column vector (2-D)
  Reshape1 : Reshape  OutputDimensionality=Column vector (2-D)
  Reshape2 : Reshape  OutputDimensionality=Column vector (2-D)
  Reshape3 : Reshape  OutputDimensionality=Customize  OutputDimensions=[3,3]
  Vector Concatenate : Concatenate  NumInputs=3
  M(i) : Outport
  wires:
  Vector Concatenate/1 -> Reshape3/1
  Constant5/1 -> Mux2/1
  Constant3/1 -> Mux2/3
  Constant4/1 -> Mux2/2
  Cos1/1 -> Multiply/1
  Constant1/1 -> Mux/1
  Cos/1 -> Mux/2
  Multiply/1 -> Mux/3
  Constant2/1 -> Mux1/1
  Cos3/1 -> Mux1/2
  Cos2/1 -> Mux1/3
  i/1 -> Cos2/1, Cos/1, Cos1/1, Cos3/1
  Mux2/1 -> Reshape/1
  Reshape/1 -> Vector Concatenate/1
  Mux/1 -> Reshape1/1
  Reshape1/1 -> Vector Concatenate/2
  Reshape2/1 -> Vector Concatenate/3
  Mux1/1 -> Reshape2/1
  Reshape3/1 -> M(i)/1

== system Main_simulation_davide/Relative attitude/A_LN/true anomaly matrix ==
  theta : Inport
  Constant{1..2,4..5} (4 alike) : Constant  Value=0
  Constant3 : Constant
  Cos : Trigonometry  Operator=cos
  Cos1 : Trigonometry
  Cos2 : Trigonometry  Operator=cos
  Cos3 : Trigonometry
  Multiply : Gain  Gain=-1
  Mux : Mux  Inputs=3
  Mux1 : Mux  Inputs=3
  Mux2 : Mux  Inputs=3
  Reshape : Reshape  OutputDimensionality=Column vector (2-D)
  Reshape1 : Reshape  OutputDimensionality=Column vector (2-D)
  Reshape2 : Reshape  OutputDimensionality=Column vector (2-D)
  Reshape3 : Reshape  OutputDimensionality=Customize  OutputDimensions=[3,3]
  Vector Concatenate : Concatenate  NumInputs=3
  M(theta) : Outport
  wires:
  Multiply/1 -> Mux/2
  Cos/1 -> Mux/1
  Constant1/1 -> Mux/3
  Constant2/1 -> Mux1/3
  theta/1 -> Cos/1, Cos1/1, Cos3/1, Cos2/1
  Vector Concatenate/1 -> Reshape3/1
  Cos3/1 -> Mux1/1
  Constant5/1 -> Mux2/1
  Cos2/1 -> Mux1/2
  Constant3/1 -> Mux2/3
  Constant4/1 -> Mux2/2
  Cos1/1 -> Multiply/1
  Mux/1 -> Reshape/1
  Reshape/1 -> Vector Concatenate/1
  Reshape1/1 -> Vector Concatenate/2
  Mux1/1 -> Reshape1/1
  Mux2/1 -> Reshape2/1
  Reshape2/1 -> Vector Concatenate/3
  Reshape3/1 -> M(theta)/1

== system Main_simulation_davide/Attitude determination/Attitude determination/q to DCM/q_cross ==
  q_vect : Inport
  Demux : Demux  Outputs=3
  Gain : Gain  Gain=-1
  Gain1 : Gain  Gain=-1
  Gain2 : Gain  Gain=-1
  Ground : Ground
  Reshape : Reshape  OutputDimensionality=Customize  OutputDimensions=[3,3]
  Vector Concatenate : Concatenate  NumInputs=9
  q_cross : Outport
  wires:
  q_vect/1 -> Demux/1
  Reshape/1 -> q_cross/1
  Vector Concatenate/1 -> Reshape/1
  Ground/1 -> Vector Concatenate/1, Vector Concatenate/5, Vector Concatenate/9
  Gain/1 -> Vector Concatenate/3
  Gain1/1 -> Vector Concatenate/4
  Gain2/1 -> Vector Concatenate/8
  Demux/1 -> [q1]
  Demux/2 -> [q2]
  Demux/3 -> [q3]
  [q3] -> Vector Concatenate/2
  [q2] -> Gain/1
  [q3] -> Gain1/1
  [q1] -> Vector Concatenate/6
  [q2] -> Vector Concatenate/7
  [q1] -> Gain2/1

== system Main_simulation_davide/Attitude determination/Sensors/Magnetometer/Magnetometer  ==
  A_BN : Inport
  Error Matrices : Subsystem
  Matrix Multiply : Product  Inputs=4  Multiplication=Matrix(*)
  RC Low Pass FIlter : Subsystem
  orthonormalization step 1 : Subsystem
  orthonormalization step 2 : Subsystem
  orthonormalization step 3 : Subsystem
  A_BN*_filtered : Outport
  wires:
  A_BN/1 -> Matrix Multiply/1
  Matrix Multiply/1 -> RC Low Pass FIlter/1(A*)
  Error Matrices/1(A_no) -> Matrix Multiply/2
  Error Matrices/2(A_sf) -> Matrix Multiply/3
  Error Matrices/3(A_noise) -> Matrix Multiply/4
  orthonormalization step 1/1(A_BN*_filtered) -> orthonormalization step 2/1(A*(t))
  RC Low Pass FIlter/1(A*_filtered) -> orthonormalization step 1/1(A*(t))
  orthonormalization step 2/1(A_BN*_filtered) -> orthonormalization step 3/1(A*(t))
  orthonormalization step 3/1(A_BN*_filtered) -> A_BN*_filtered/1

== system Main_simulation_davide/Attitude determination/Sensors/Magnetometer/b_B computation ==
  A_BN* : Inport
  b_N : Inport  Port=2
  Matrix Multiply : Product  Multiplication=Matrix(*)
  Saturation : Subsystem
  b_B : Outport
  wires:
  A_BN*/1 -> Matrix Multiply/1
  b_N/1 -> Matrix Multiply/2
  Matrix Multiply/1 -> Saturation/1(b_B)
  Saturation/1(b_B saturated) -> b_B/1

== system Main_simulation_davide/Attitude determination/Sensors/Magnetometer/model to reality difference ==
  A_BN : Inport
  A_BN* : Inport  Port=2
  b_N : Inport  Port=3
  MatrixMultiply : Product  Multiplication=Matrix(*)
  MatrixMultiply1 : Product  Multiplication=Matrix(*)
  Scope : Scope
  Sum : Sum  Inputs=|-|+|
  wires:
  A_BN*/1 -> MatrixMultiply/1
  b_N/1 -> MatrixMultiply1/2, MatrixMultiply/2
  A_BN/1 -> MatrixMultiply1/1
  MatrixMultiply1/1 -> Sum/1
  MatrixMultiply/1 -> Sum/2
  Sum/1 -> Scope/1

== system Main_simulation_davide/Control/Slew/Desired attitude/orthonormalization step 1 ==
  A*(t) : Inport
  Gain : Gain  Gain=3/2
  Gain1 : Gain  Gain=1/2
  Matrix Multiply : Product  Inputs=3  Multiplication=Matrix(*)
  Sum : Sum  Inputs=-+
  Transpose : Math  Operator=transpose  SaturateOnIntegerOverflow=on
  A_BN*_filtered : Outport
  wires:
  A*(t)/1 -> Transpose/1, Gain1/1, Matrix Multiply/1, Gain/1
  Sum/1 -> A_BN*_filtered/1
  Gain/1 -> Sum/2
  Transpose/1 -> Matrix Multiply/2
  Gain1/1 -> Matrix Multiply/3
  Matrix Multiply/1 -> Sum/1

== system Main_simulation_davide/Enviroment/Solar radiation/Force MB/Subsystem ==
  S_B : Inport
  N_MB : Inport  Port=2
  Constant3 : Constant  Value=[1, 1, 1]
  Matrix Multiply5 : Product  Multiplication=Matrix(*)
  Product10 : Product
  Reshape11 : Reshape  OutputDimensionality=Row vector (2-D)
  Reshape12 : Reshape  OutputDimensionality=Column vector (2-D)
  Sum of Elements : Sum  Inputs=+  CollapseMode=Specified dimension  CollapseDim=2
  Out1 : Outport
  wires:
  Matrix Multiply5/1 -> Product10/1
  Reshape12/1 -> Matrix Multiply5/1
  S_B/1 -> Reshape12/1
  Product10/1 -> Sum of Elements/1
  N_MB/1 -> Product10/2
  Sum of Elements/1 -> Out1/1
  Constant3/1 -> Reshape11/1
  Reshape11/1 -> Matrix Multiply5/2

== system Main_simulation_davide/Enviroment/Solar radiation/S_B dot N_MB/If Action Subsystem ==
  NMB : Inport
  Action Port : ActionPort  ActionPortLabel=if(u1 > 0)
  Constant : Constant
  Selector : Selector  NumberOfDimensions=2  InputPortWidth=3  IndexOptions=Index vector (dialog),Index vector (dialog)  Indices=1,[1 2 3]  OutputSizes=1,1
  x : Outport
  pointer : Outport  Port=2
  wires:
  NMB/1 -> Selector/1
  Selector/1 -> x/1
  Constant/1 -> pointer/1

== system Main_simulation_davide/Enviroment/Solar radiation/S_B dot N_MB/If Action Subsystem1 ==
  NMB : Inport
  Action Port : ActionPort  ActionPortLabel=if(u1 > 0)
  Constant : Constant
  Selector : Selector  NumberOfDimensions=2  InputPortWidth=3  IndexOptions=Index vector (dialog),Index vector (dialog)  Indices=2,[1 2 3]  OutputSizes=1,1
  y : Outport
  pointer : Outport  Port=2
  wires:
  Selector/1 -> y/1
  NMB/1 -> Selector/1
  Constant/1 -> pointer/1

== system Main_simulation_davide/Enviroment/Solar radiation/S_B dot N_MB/If Action Subsystem2 ==
  NMB : Inport
  Action Port : ActionPort  ActionPortLabel=if(u1 > 0)
  Constant : Constant
  Selector : Selector  NumberOfDimensions=2  InputPortWidth=3  IndexOptions=Index vector (dialog),Index vector (dialog)  Indices=3,[1 2 3]  OutputSizes=1,1
  z : Outport
  pointer : Outport  Port=2
  wires:
  NMB/1 -> Selector/1
  Selector/1 -> z/1
  Constant/1 -> pointer/1

== system Main_simulation_davide/Enviroment/Solar radiation/S_B dot N_MB/If Action Subsystem3 ==
  NMB : Inport
  Action Port : ActionPort  ActionPortLabel=else
  Constant : Constant  Value=-1
  Selector : Selector  NumberOfDimensions=2  InputPortWidth=3  IndexOptions=Index vector (dialog),Index vector (dialog)  Indices=4,[1 2 3]  OutputSizes=1,1
  -x : Outport
  pointer : Outport  Port=2
  wires:
  Selector/1 -> -x/1
  NMB/1 -> Selector/1
  Constant/1 -> pointer/1

== system Main_simulation_davide/Enviroment/Solar radiation/S_B dot N_MB/If Action Subsystem4 ==
  NMB : Inport
  Action Port : ActionPort  ActionPortLabel=else
  Constant : Constant  Value=-1
  Selector : Selector  NumberOfDimensions=2  InputPortWidth=3  IndexOptions=Index vector (dialog),Index vector (dialog)  Indices=5,[1 2 3]  OutputSizes=1,1
  -y : Outport
  pointer : Outport  Port=2
  wires:
  NMB/1 -> Selector/1
  Selector/1 -> -y/1
  Constant/1 -> pointer/1

== system Main_simulation_davide/Enviroment/Solar radiation/S_B dot N_MB/If Action Subsystem5 ==
  NMB : Inport
  Action Port : ActionPort  ActionPortLabel=else
  Constant : Constant  Value=-1
  Selector : Selector  NumberOfDimensions=2  InputPortWidth=3  IndexOptions=Index vector (dialog),Index vector (dialog)  Indices=6,[1 2 3]  OutputSizes=1,1
  -z : Outport
  pointer : Outport  Port=2
  wires:
  Selector/1 -> -z/1
  NMB/1 -> Selector/1
  Constant/1 -> pointer/1

== system Main_simulation_davide/Enviroment/Solar radiation/S_B dot N_SP/If Action Subsystem ==
  N_SP : Inport
  Action Port : ActionPort  ActionPortLabel=if(u1 > 0)
  Constant : Constant
  Selector : Selector  NumberOfDimensions=2  InputPortWidth=3  IndexOptions=Index vector (dialog),Index vector (dialog)  Indices=1,[1 2 3]  OutputSizes=1,1
  true_NSP : Outport
  pointer : Outport  Port=2
  wires:
  N_SP/1 -> Selector/1
  Constant/1 -> pointer/1
  Selector/1 -> true_NSP/1

== system Main_simulation_davide/Enviroment/Solar radiation/S_B dot N_SP/If Action Subsystem1 ==
  N_SP : Inport
  Action Port : ActionPort  ActionPortLabel=if(u1 > 0)
  Constant : Constant  Value=-1
  Selector : Selector  NumberOfDimensions=2  InputPortWidth=3  IndexOptions=Index vector (dialog),Index vector (dialog)  Indices=2,[1 2 3]  OutputSizes=1,1
  true_NSP : Outport
  pointer : Outport  Port=2
  wires:
  Selector/1 -> true_NSP/1
  Constant/1 -> pointer/1
  N_SP/1 -> Selector/1
